simulink model "lab3_sim"  (R2025b)
settings: Solver=VariableStepAuto  StartTime=0.0  StopTime=Tend  RelTol=1e-3
values from neighbouring files (symbols this model uses):
  delta_1 = 0    [lab3.m]
  delta_2 = 1    [lab3.m]
  rho = 0    [lab3.m]
  Ts = 0.01    [lab3.m]
undefined symbols (not defined in the file or in its folder): DiscIntNeverNeededParam
libraries: cstblocks x2
settings Model: Creator=davidecovolo  LastModifiedBy=davidecovolo

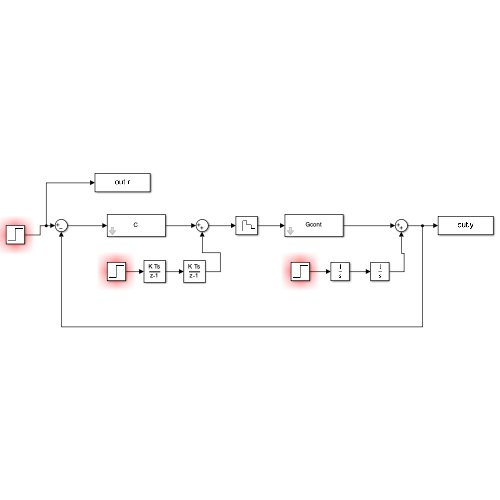
[thumbnail: Simulink's stored preview of the top-level diagram]
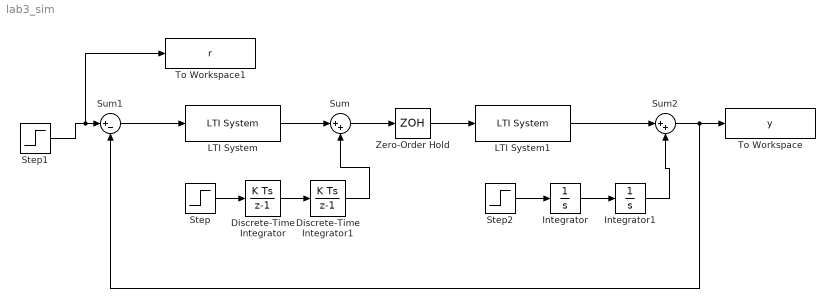
== system lab3_sim ==
  Discrete-Time Integrator : DiscreteIntegrator  SampleTime=Ts  ICPrevOutput=DiscIntNeverNeededParam  ICPrevScaledInput=DiscIntNeverNeededParam
  Discrete-Time Integrator1 : DiscreteIntegrator  SampleTime=Ts  ICPrevOutput=DiscIntNeverNeededParam  ICPrevScaledInput=DiscIntNeverNeededParam
  Integrator : Integrator
  Integrator1 : Integrator
  LTI System : cstblocks/LTI System  sys=C  IC=[]  PadeOrder=0
  LTI System1 : cstblocks/LTI System  sys=Gcont  IC=[]  PadeOrder=0
  Step : Step  Time=0  After=delta_1  SampleTime=0
  Step1 : Step  Time=0  After=rho  SampleTime=0
  Step2 : Step  Time=0  After=delta_2  SampleTime=0
  Sum : Sum  Inputs=|++
  Sum1 : Sum  Inputs=|+-
  Sum2 : Sum  Inputs=|++
  To Workspace : ToWorkspace  VariableName=y  SaveFormat=Timeseries  SampleTime=-1
  To Workspace1 : ToWorkspace  VariableName=r  SaveFormat=Timeseries  SampleTime=-1
  Zero-Order Hold : ZeroOrderHold  SampleTime=Ts
  wires:
  Zero-Order Hold/1 -> LTI System1/1
  Step2/1 -> Integrator/1
  Integrator/1 -> Integrator1/1
  Integrator1/1 -> Sum2/2
  Discrete-Time Integrator/1 -> Discrete-Time Integrator1/1
  Step/1 -> Discrete-Time Integrator/1
  Discrete-Time Integrator1/1 -> Sum/2
  LTI System/1 -> Sum/1
  Sum/1 -> Zero-Order Hold/1
  LTI System1/1 -> Sum2/1
  Sum2/1 -> To Workspace/1, Sum1/2
  Step1/1 -> To Workspace1/1, Sum1/1
  Sum1/1 -> LTI System/1
